simulink model "EnergyManSyst"  (R2019b)
settings: Solver=VariableStepAuto  StartTime=0.0  StopTime=8760  RelTol=1e-3
undefined symbols (not defined in the file): GHI, K1, K2, K3, K4, tempreture, time
libraries: simulink x4
settings Model: Creator=HP  LastModifiedBy=HP

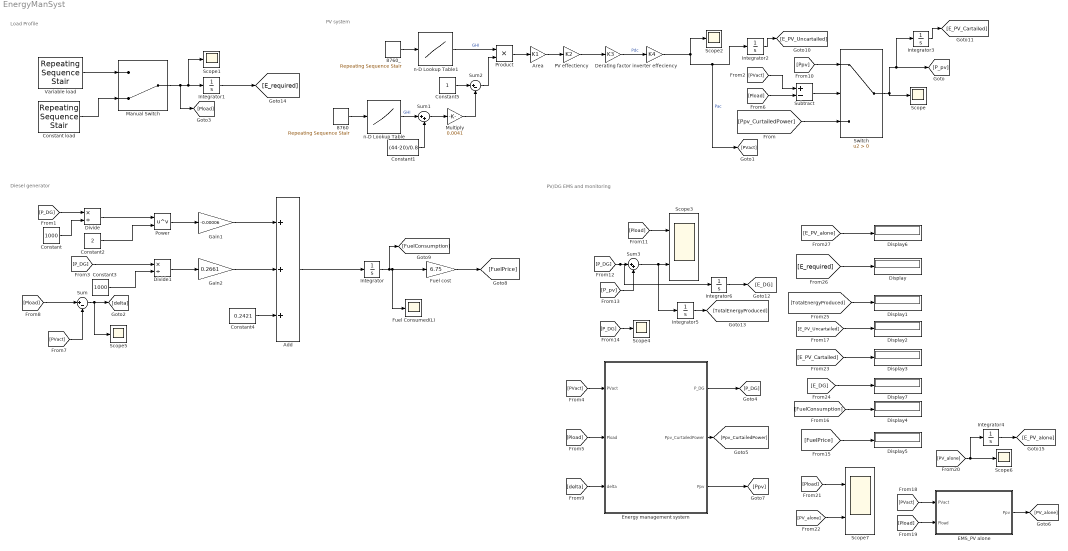
== system EnergyManSyst ==
  note: PV/DG EMS and monitoring
  note: Load Profile
  note: Diesel generator
  note: PV system
  8760 : simulink/Sources/Repeating Sequence Stair  OutValues=time  tsamp=1  OutMin=[]  OutMax=[]  OutDataTypeStr=double  OutputDataTypeScalingMode=double  OutDataType=fixdt(0,8)  ConRadixGroup=Best Precision: Vector-wise  OutScaling=2^-12
  8760_ : simulink/Sources/Repeating Sequence Stair  OutValues=time  tsamp=1  OutMin=[]  OutMax=[]  OutDataTypeStr=double  OutputDataTypeScalingMode=double  OutDataType=fixdt(0,8)  ConRadixGroup=Best Precision: Vector-wise  OutScaling=2^-12
  Add : Sum  Inputs=+++
  Area : Gain  Gain=K1
  Constant : Constant  Value=1000
  Constant load : simulink/Sources/Repeating Sequence Stair  OutValues=constantload  tsamp=1  OutMin=[]  OutMax=[]  OutDataTypeStr=double  OutputDataTypeScalingMode=double  OutDataType=fixdt(0,8)  ConRadixGroup=Best Precision: Vector-wise  OutScaling=2^-12
  Constant1 : Constant  Value=(44-20)/0.8
  Constant2 : Constant  Value=2
  Constant3 : Constant  Value=1000
  Constant4 : Constant  Value=0.2421
  Constant5 : Constant
  "Derating factor  " : Gain  Gain=K3
  Display{,1..7} (8 alike) : Display
  Divide : Product  Inputs=*/
  Divide1 : Product  Inputs=*/
  EMS_PV alone : MATLAB Function  TreatAsAtomicUnit=on
  Energy management system : MATLAB Function  TreatAsAtomicUnit=on
  Fuel Consumed(L) : Scope
  Fuel cost : Gain  Gain=6.75
  Gain1 : Gain  Gain=-0.00006
  Gain2 : Gain  Gain=0.2661
  Integrator{,1..6} (7 alike) : Integrator
  Manual Switch : ManualSwitch  CurrentSetting=0
  Multiply : Gain  Gain=0.0041
  PV effectiency : Gain  Gain=K2
  Power : Math  Operator=pow  SignedPower=off  SaturateOnIntegerOverflow=on
  Product : Product
  Scope{,1..2,4..6} (6 alike) : Scope
  Scope3 : Scope  NumInputPorts=2
  Scope7 : Scope  NumInputPorts=2
  Subtract : Sum  Inputs=+-
  Sum : Sum  Inputs=|+-
  Sum1 : Sum  Inputs=|++
  Sum2 : Sum  Inputs=|+-
  Sum3 : Sum  Inputs=|++
  Switch : Switch  Criteria=u2 > Threshold
  Variable load : simulink/Sources/Repeating Sequence Stair  OutValues=load  tsamp=1  OutMin=[]  OutMax=[]  OutDataTypeStr=double  OutputDataTypeScalingMode=double  OutDataType=fixdt(0,8)  ConRadixGroup=Best Precision: Vector-wise  OutScaling=2^-12
  inverter effeciency : Gain  Gain=K4
  n-D Lookup Table : Lookup_n-D  NumberOfTableDimensions=1  BreakpointsForDimension1=time  BreakpointsForDimension3=[5, 7]  Table=tempreture  InternalRulePriority=Speed  RndMeth=Simplest  InputSameDT=on
  n-D Lookup Table1 : Lookup_n-D  NumberOfTableDimensions=1  BreakpointsForDimension1=time  BreakpointsForDimension3=[5, 7]  Table=GHI  InternalRulePriority=Speed  RndMeth=Simplest  InputSameDT=on
  wires:
  8760/1 -> n-D Lookup Table/1
  PV effectiency/1 -> "Derating factor  "/1
  "Derating factor  "/1 -> inverter effeciency/1  "Pdc"
  Area/1 -> PV effectiency/1
  Constant4/1 -> Add/3
  Fuel cost/1 -> [FuelPrice]
  [P_DG] -> Divide/1
  Divide1/1 -> Gain2/1
  Constant3/1 -> Divide1/2
  Add/1 -> Integrator/1
  Constant2/1 -> Power/2
  Gain1/1 -> Add/1
  Constant/1 -> Divide/2
  Gain2/1 -> Add/2
  [P_DG] -> Divide1/1
  Divide/1 -> Power/1
  Power/1 -> Gain1/1
  Integrator/1 -> [FuelConsumption], Fuel cost/1, Fuel Consumed(L)/1
  [PVact] -> Energy management system/1(PVact)
  [Pload] -> Energy management system/2(Pload)
  Energy management system/1(P_DG) -> [P_DG]
  Energy management system/2(Ppv_CurtailedPower) -> [Ppv_CurtailedPower]
  [PVact] -> Subtract/1
  [Pload] -> Subtract/2
  [Ppv_CurtailedPower] -> Switch/3
  Subtract/1 -> Switch/2
  Sum/1 -> Scope5/1, [delta]
  [delta] -> Energy management system/3(delta)
  Integrator1/1 -> [E_required]
  Integrator2/1 -> [E_PV_Uncartailed]
  n-D Lookup Table/1 -> Sum1/1  "GHI"
  Constant1/1 -> Sum1/2
  Sum1/1 -> Multiply/1
  Constant5/1 -> Sum2/1
  Multiply/1 -> Sum2/2
  8760_/1 -> n-D Lookup Table1/1
  n-D Lookup Table1/1 -> Product/1  "GHI"
  Sum2/1 -> Product/2
  Product/1 -> Area/1
  inverter effeciency/1 -> Scope2/1, Integrator2/1, [PVact]  "Pac"
  Switch/1 -> Integrator3/1, [P_pv], Scope/1
  Energy management system/3(Ppv) -> [Ppv]
  [Ppv] -> Switch/1
  [Pload] -> Scope3/1
  [P_DG] -> Integrator6/1, Sum3/1
  [P_pv] -> Sum3/2
  [P_DG] -> Scope4/1
  [Pload] -> Sum/1
  Integrator5/1 -> [TotalEnergyProduced]
  Sum3/1 -> Integrator5/1, Scope3/2
  Variable load/1 -> Manual Switch/1
  Constant load/1 -> Manual Switch/2
  Manual Switch/1 -> [Pload], Scope1/1, Integrator1/1
  EMS_PV alone/1(Ppv) -> [PV_alone]
  [PVact] -> EMS_PV alone/1(PVact)
  [Pload] -> EMS_PV alone/2(Pload)
  [PV_alone] -> Integrator4/1, Scope6/1
  Integrator4/1 -> [E_PV_alone]
  [Pload] -> Scope7/1
  [PV_alone] -> Scope7/2
  [PVact] -> Sum/2
  Integrator6/1 -> [E_DG]
  Integrator3/1 -> [E_PV_Cartailed]
  [E_required] -> Display/1
  [TotalEnergyProduced] -> Display1/1
  [E_PV_Uncartailed] -> Display2/1
  [E_PV_Cartailed] -> Display3/1
  [FuelConsumption] -> Display4/1
  [FuelPrice] -> Display5/1
  [E_PV_alone] -> Display6/1
  [E_DG] -> Display7/1

== matlab function EnergyManSyst/Energy management system ==
  data: PVact input; P_DG output; Pload input; Ppv_CurtailedPower output; delta input; Ppv output
function [P_DG, Ppv_CurtailedPower, Ppv]= EMS(PVact, Pload, delta)
Ppv_CurtailedPower = 0;
P_DG = 0;
P_DGrated = 1500;
P_DGmin= P_DGrated*0.25;
Ppv = 0;

if PVact > Pload
    if  Pload == 0
        Ppv = 0;
        P_DG = 0;
    end
    Ppv = Pload;
    P_DG =0;
end



if PVact<Pload
    if delta < P_DGmin
        %%Curtailment needed
        %if PVact > P_DGmin
        Ppv_CurtailedPower = PVact - P_DGmin; 
        %end
        P_DG = P_DGmin;
    end
    
    if delta > P_DGmin 
       P_DG = Pload - PVact;
       if P_DG > P_DGrated
          P_DG = P_DGrated;
       elseif P_DG < P_DGmin 
           P_DG = P_DGmin;
       end 
       Ppv_CurtailedPower = PVact;
    end
end
end

== matlab function EnergyManSyst/EMS_PV alone ==
  data: PVact input; Ppv output; Pload input
function Ppv = EMS_PV(PVact, Pload)
Ppv = 0;
if PVact > Pload
    if  Pload == 0
        Ppv = 0;
    end
    Ppv = Pload;
    if PVact > 1.02* Pload
    Ppv = 1.02*Pload;
    end
else
    Ppv = PVact;
end
